simulink model "curiosity_i2c_pitch_roll"  (R2024b)
settings: Solver=FixedStepDiscrete  StartTime=0.0  StopTime=inf  FixedStep=1e-3  RelTol=1e-3  EnableMultiTasking=on
undefined symbols (not defined in the file): A0, ADC, D10, D7, D8, D9, DiscIntNeverNeededParam, Max, MaxPer, ms, NumBits1, NumBits2, P1, P58, P59, Pin, Resol, s, Timer, us
libraries: MCHP_Blockset x18, simulink x15, dspstat3 x1
(part 1 of 4)
settings Model: SimulationMode=external  ExtModeEnableFloating=off  ExtModeTrigDuration=20  Creator=I52209  LastModifiedBy=I67977
settings SolverCC: AlgebraicLoopSolver=TrustRegion
settings OptimizationCC: DefaultUnderspecifiedDataType=single  EnhancedBackFolding=on  BooleansAsBitfields=on  PassReuseOutputArgsAs=Individual arguments  ZeroExternalMemoryAtStartup=off  ZeroInternalMemoryAtStartup=off  OptimizeBlockOrder=speed  DifferentSizesBufferReuse=on  EfficientTunableParamExpr=on
settings DebuggingCC: MultiTaskDSMMsg=none  MultiTaskCondExecSysMsg=none  MultiTaskRateTransMsg=warning  ParameterTunabilityLossMsg=error  ArithmeticOperatorsInVariantConditions=warning
settings HardwareCC: ProdBitPerPointer=32  ProdBitPerSizeT=32  ProdBitPerPtrDiffT=32  ProdLargestAtomicInteger=Long  ProdWordSize=32  ProdLongLongMode=on  ProdHWDeviceType=Generic->Custom
settings ModelReferenceCC: ModelReferenceNumInstancesAllowed=Single
settings SFSimCC: MATLABDynamicMemAlloc=off  CustomCodeUndefinedFunction=UseInterfaceOnly
settings RTWCC: Description=Microchip Embedded Target dsPIC33A (real-time)  SystemTargetFile=MCHP_dsPIC33A_stf.tlc  TLCOptions="-aExtModeXCPClassicInterface=0  -aCreateExtModeTypes=1 -aExtModeXCPSimulationTimeInTicks=1"  TemplateMakefile=MCHP_dsPIC33A.tmf  GPUComputeCapability=3.5
settings CodeAppCC: ForceParamTrailComments=on  IgnoreCustomStorageClasses=off  MaxIdLength=255  OperatorAnnotations=on  SimulinkDataObjDesc=on  SFDataObjDesc=on  InsertBlockDesc=on
settings STFCustomTargetCC: TargetLibSuffix=_lib.a  TargetLangStandard=C99 (ISO)  MultiwordLength=256  CombineOutputUpdateFcns=on  CombineSignalStateStructs=on  ERTCustomFileBanners=on  SupportContinuousTime=off  RemoveResetFunc=on  MATLABClassNameForMDSCustomization=Simulink.SoftwareTarget.ERTCustomization  SystemTargetFile=MCHP_dsPIC33A_stf.tlc
settings ERTTargetCC: TargetLibSuffix=_lib.a  TargetLangStandard=C99 (ISO)  ParMdlRefBuildCompliant=off  CompOptLevelCompliant=off  ConcurrentExecutionCompliant=off  CombineSignalStateStructs=on  SupportNonInlinedSFcns=on  ModelStepFunctionPrototypeControlCompliant=off  CPPClassGenCompliant=off  UseToolchainInfoCompliant=off  ExtMode=on  ExtModeTransport=1  ExtModeStaticAlloc=on  ExtModeStaticAllocSize=2048  ExtModeMexFile=ext_xcp  ExtModeMexArgs=1 52 460800 './curiosity_i2c.X/curiosity_i2c.elf'  ExtModeIntrfLevel=Level2 - Open  InlinedParameterPlacement=Hierarchical  ERTSrcFileBannerTemplate=MCHP_dsPIC_code_template.cgt  ERTHdrFileBannerTemplate=MCHP_dsPIC_code_template.cgt  ERTDataSrcFileTemplate=MCHP_dsPIC_code_template.cgt  ERTDataHdrFileTemplate=MCHP_dsPIC_code_template.cgt  ERTCustomFileTemplate=MCHP_main.tlc  MaxLineWidth=110  DynamicArrayContainerType=coder::array

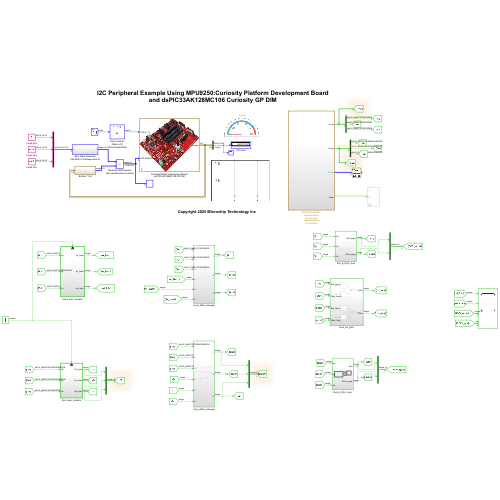
[thumbnail: Simulink's stored preview of the top-level diagram]
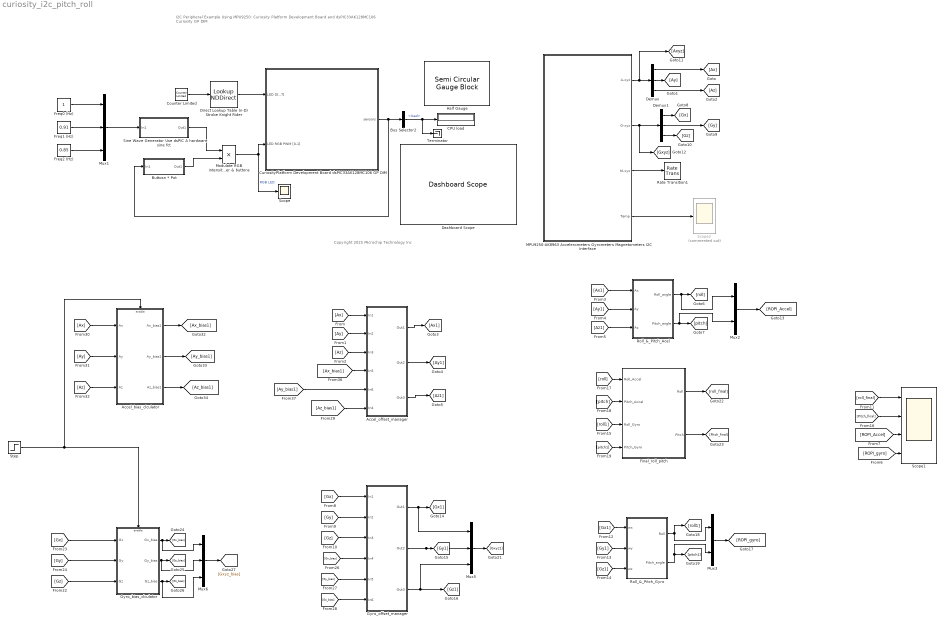
== system curiosity_i2c_pitch_roll ==
  note: I2C Peripheral Example Using MPU9250: Curiosity Platform Development Board and dsPIC33AK128MC106 Curiosity GP DIM
  note: Copyright 2025 Microchip Technology Inc
  Accel_bias_clculator : Subsystem  TreatAsAtomicUnit=on
  Accel_offset_manager : Subsystem
  Bus Selector2 : BusSelector  OutputSignals=MCU.load
  Buttosn * Pot : Subsystem
  CPU load : Display
  Counter Limited : simulink/Sources/Counter Limited  uplimit=13  tsamp=0.05
  CuriosityPlatform Development Board dsPIC33AK128MC106 GP DIM : Subsystem
      mask Display: image('MCHP_i_Board_Curiosity_dsPICA.jpg')
  Dashboard Scope : DashboardScope  TimeSpan=5  Ymin=0  Ymax=1  LegendPosition=Hide  ScaleAtStop=off  TicksPosition=Inside
  Demux : Demux  Outputs=3
  Demux1 : Demux  Outputs=3
  Direct Lookup Table (n-D) Strobe Knight Rider : LookupNDDirect  NumberOfTableDimensions=1  Table=uint16(2.^[[0:7] [6:-1:1]] )  RemoveProtectionInput=on
  Final_roll_pitch : Subsystem
  Freq0 (Hz) : Constant  OutDataTypeStr=fixdt(0,16,10)
  Freq1 (Hz) : Constant  Value=0.91  OutDataTypeStr=fixdt(0,16,10)
  Freq2 (Hz) : Constant  Value=0.85  OutDataTypeStr=fixdt(0,16,10)
  Gyro_bias_clculator : Subsystem  TreatAsAtomicUnit=on
  Gyro_offset_manager : Subsystem
  Half Gauge : SemiCircularGaugeBlock
  MPU9250-AK8963 Accelerometers Gyrometers Magnetometers I2C Interface : Subsystem
  Modulate RGB intensity with potentiometer & buttons : Product  OutDataTypeStr=single
  Mux1 : Mux  Inputs=3
  Mux2 : Mux  Inputs=2
  Mux3 : Mux  Inputs=2
  Mux5 : Mux  Inputs=3
  Mux6 : Mux  Inputs=3
  Rate Transition1 : RateTransition  Deterministic=off  OutPortSampleTimeOpt=Inherit
  Roll_&_Pitch_Acel : Subsystem
  Roll_&_Pitch_Gyro : Subsystem
  Scope : Scope
  Scope1 : Scope  NumInputPorts=4
  Scope2 : Scope  Commented=on
  Sine Wave Generator Use dsPIC A hardware sine fct : Subsystem
  Step : Step  Time=2  Before=1  After=0  SampleTime=0.005
  Terminator : Terminator
  wires:
  Buttosn * Pot/1(Out1) -> Modulate RGB intensity with potentiometer & buttons/2
  Bus Selector2/1 -> Terminator/1, CPU load/1  "<load>"
  Sine Wave Generator Use dsPIC A hardware sine fct/1(Out1) -> Modulate RGB intensity with potentiometer & buttons/1
  Mux1/1 -> Sine Wave Generator Use dsPIC A hardware sine fct/1(In1)
  Freq0 (Hz)/1 -> Mux1/1
  Freq1 (Hz)/1 -> Mux1/2
  Freq2 (Hz)/1 -> Mux1/3
  Direct Lookup Table (n-D) Strobe Knight Rider/1 -> CuriosityPlatform Development Board dsPIC33AK128MC106 GP DIM/1(LED [0...7])
  Modulate RGB intensity with potentiometer & buttons/1 -> CuriosityPlatform Development Board dsPIC33AK128MC106 GP DIM/2(LED RGB PWM [0-1]), Scope/1  "RGB LED"
  CuriosityPlatform Development Board dsPIC33AK128MC106 GP DIM/1(sensors) -> Buttosn * Pot/1(In1), Bus Selector2/1
  Counter Limited/1 -> Direct Lookup Table (n-D) Strobe Knight Rider/1
  MPU9250-AK8963 Accelerometers Gyrometers Magnetometers I2C Interface/1(A-xyz) -> Demux/1, [Axyz]
  Demux1/2 -> [Gy]
  MPU9250-AK8963 Accelerometers Gyrometers Magnetometers I2C Interface/2(G-xyz) -> [Gxyz], Demux1/1
  MPU9250-AK8963 Accelerometers Gyrometers Magnetometers I2C Interface/3(M-xyz) -> Rate Transition1/1
  MPU9250-AK8963 Accelerometers Gyrometers Magnetometers I2C Interface/4(Temp) -> Scope2/1
  Demux/1 -> [Ax]
  Demux/2 -> [Ay]
  Demux/3 -> [Az]
  Demux1/1 -> [Gx]
  Demux1/3 -> [Gz]
  [Gy] -> Gyro_offset_manager/2(In2)
  [Gy] -> Gyro_bias_clculator/2(Gy)
  Accel_offset_manager/2(Out2) -> [Ay1]
  [Ax] -> Accel_bias_clculator/1(Ax)
  Roll_&_Pitch_Acel/1(Roll_angle) -> Mux2/1, [roll]
  [Gx] -> Gyro_bias_clculator/1(Gx)
  [Ay] -> Accel_offset_manager/2(In2)
  [Az_bias1] -> Accel_offset_manager/6(In4)
  [ROPI_Accel] -> Scope1/3
  Final_roll_pitch/2(Pitch) -> [Pitch_final]
  [Ax1] -> Roll_&_Pitch_Acel/1(Ax)
  Gyro_offset_manager/2(Out2) -> Mux5/2, [Gy1]
  Mux6/1 -> [Gxyz_bias]
  [Az1] -> Roll_&_Pitch_Acel/3(Az)
  Gyro_bias_clculator/2(Gy_bias) -> Mux6/2, [Gy_bias]
  [Gx] -> Gyro_offset_manager/1(In1)
  [roll] -> Final_roll_pitch/1(Roll_Accel)
  [Az] -> Accel_offset_manager/3(In3)
  [Gz] -> Gyro_bias_clculator/3(Gz)
  [Gx1] -> Roll_&_Pitch_Gyro/1(wx)
  [roll1] -> Final_roll_pitch/3(Roll_Gyro)
  Roll_&_Pitch_Gyro/2(Pitch_angle) -> Mux3/2, [pitch1]
  Gyro_offset_manager/1(Out1) -> [Gx1], Mux5/1
  [Ay_bias1] -> Accel_offset_manager/5(In6)
  Mux2/1 -> [ROPI_Accel]
  [Gx_bias] -> Gyro_offset_manager/4(In4)
  [Ay1] -> Roll_&_Pitch_Acel/2(Ay)
  Final_roll_pitch/1(Roll) -> [roll_final]
  Step/1 -> Accel_bias_clculator/Enable, Gyro_bias_clculator/Enable
  Mux3/1 -> [ROPI_gyro]
  [pitch] -> Final_roll_pitch/2(Pitch_Accel)
  Accel_bias_clculator/2(Ay_bias1) -> [Ay_bias1]
  [Gz] -> Gyro_offset_manager/3(In3)
  Accel_bias_clculator/3(Az_bias1) -> [Az_bias1]
  Accel_offset_manager/1(Out1) -> [Ax1]
  Gyro_offset_manager/3(Out3) -> Mux5/3, [Gz1]
  Gyro_bias_clculator/1(Gx_bias) -> Mux6/1, [Gx_bias]
  [Gz_bias] -> Gyro_offset_manager/6(In6)
  [Gy1] -> Roll_&_Pitch_Gyro/2(wy)
  [Pitch_final] -> Scope1/2
  [ROPI_gyro] -> Scope1/4
  [pitch1] -> Final_roll_pitch/4(Pitch_Gyro)
  [Ay] -> Accel_bias_clculator/2(Ay)
  [Ax] -> Accel_offset_manager/1(In1)
  [roll_final] -> Scope1/1
  Mux5/1 -> [Gxyz1]
  Gyro_bias_clculator/3(Gz_bias) -> Mux6/3, [Gz_bias]
  Roll_&_Pitch_Acel/2(Pitch_angle) -> Mux2/2, [pitch]
  Accel_bias_clculator/1(Ax_bias1) -> [Ax_bias1]
  [Ax_bias1] -> Accel_offset_manager/4(In5)
  [Gy_bias] -> Gyro_offset_manager/5(In5)
  [Az] -> Accel_bias_clculator/3(Az)
  Accel_offset_manager/3(Out3) -> [Az1]
  Roll_&_Pitch_Gyro/1(Roll) -> [roll1], Mux3/1
  [Gz1] -> Roll_&_Pitch_Gyro/3(wz)

== system curiosity_i2c_pitch_roll/Accel_bias_clculator ==
  Ax : Inport
  Ay : Inport  Port=2
  Az : Inport  Port=3
  Enable : EnablePort
  manu_mean : Subsystem
  manu_mean3 : Subsystem
  manu_mean4 : Subsystem
  Ax_bias1 : Outport
  Ay_bias1 : Outport  Port=2
  Az_bias1 : Outport  Port=3
  wires:
  Ay/1 -> manu_mean3/1(Ay)
  Ax/1 -> manu_mean/1(Ax)
  Az/1 -> manu_mean4/1(Az)
  manu_mean/1(Ax_bias1) -> Ax_bias1/1
  manu_mean3/1(Ay_bias1) -> Ay_bias1/1
  manu_mean4/1(Ax_bias1) -> Az_bias1/1

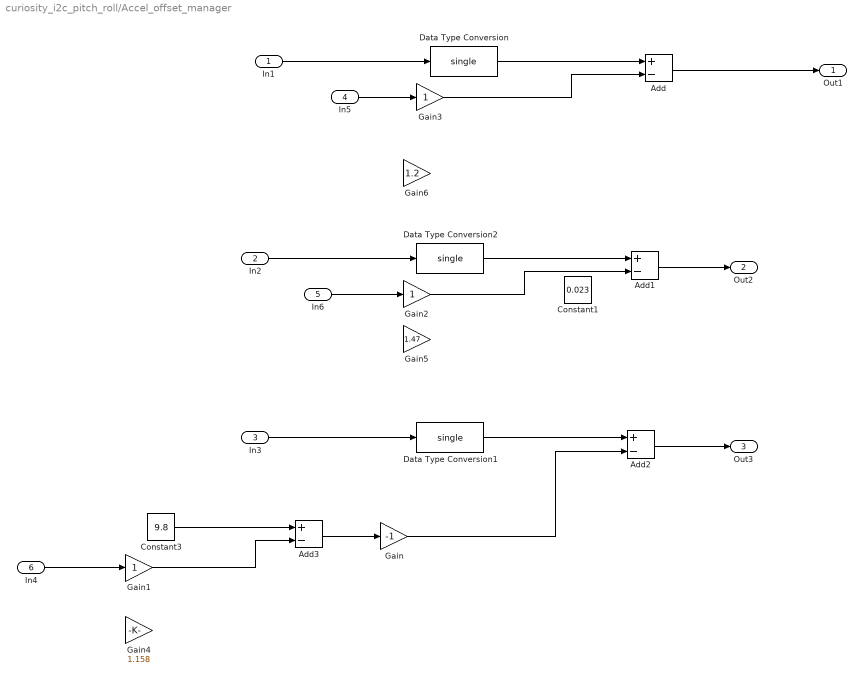
== system curiosity_i2c_pitch_roll/Accel_offset_manager ==
  In1 : Inport
  In2 : Inport  Port=2
  In3 : Inport  Port=3
  In5 : Inport  Port=4
  In6 : Inport  Port=5
  In4 : Inport  Port=6
  Add : Sum  Inputs=+-  OutDataTypeStr=Inherit: Same as first input
  Add1 : Sum  Inputs=+-  OutDataTypeStr=Inherit: Same as first input
  Add2 : Sum  Inputs=+-  OutDataTypeStr=Inherit: Same as first input
  Add3 : Sum  Inputs=+-
  Constant1 : Constant  Value=0.023  SampleTime=0.005
  Constant3 : Constant  Value=9.8  OutDataTypeStr=single  SampleTime=0.005
  Data Type Conversion : DataTypeConversion  OutDataTypeStr=single  SaturateOnIntegerOverflow=off  RndMeth=Floor
  Data Type Conversion1 : DataTypeConversion  OutDataTypeStr=single  SaturateOnIntegerOverflow=off  RndMeth=Floor
  Data Type Conversion2 : DataTypeConversion  OutDataTypeStr=single  SaturateOnIntegerOverflow=off  RndMeth=Floor
  Gain : Gain  Gain=-1
  Gain1 : Gain
  Gain2 : Gain
  Gain3 : Gain
  Gain4 : Gain  Gain=1.158
  Gain5 : Gain  Gain=1.47
  Gain6 : Gain  Gain=1.2
  Out1 : Outport
  Out2 : Outport  Port=2
  Out3 : Outport  Port=3
  wires:
  In6/1 -> Gain2/1
  Gain2/1 -> Add1/2
  Data Type Conversion2/1 -> Add1/1
  In2/1 -> Data Type Conversion2/1
  Data Type Conversion1/1 -> Add2/1
  In3/1 -> Data Type Conversion1/1
  In1/1 -> Data Type Conversion/1
  Add2/1 -> Out3/1
  Add1/1 -> Out2/1
  Data Type Conversion/1 -> Add/1
  Add/1 -> Out1/1
  Add3/1 -> Gain/1
  Constant3/1 -> Add3/1
  In4/1 -> Gain1/1
  In5/1 -> Gain3/1
  Gain3/1 -> Add/2
  Gain/1 -> Add2/2
  Gain1/1 -> Add3/2

== system curiosity_i2c_pitch_roll/Buttosn * Pot ==
  In1 : Inport
  Bus Selector : BusSelector  OutputSignals=ADC.pot
  Bus Selector1 : BusSelector  OutputSignals=BTN.S1,BTN.S2,BTN.S3
  Cast1 : DataTypeConversion  OutDataTypeStr=single  SaturateOnIntegerOverflow=off  RndMeth=Floor
  Desactivate R,G or B with buttons 1,2 or 3 multiplied by pot : Product  OutDataTypeStr=single
  Downsample x10 : Subsystem  mask{DownSample=10}
      mask prompts: DownSample "DownSample Factor"
  Mux : Mux  Inputs=3
  Rate Transition : RateTransition
  Out1 : Outport
  wires:
  Mux/1 -> Cast1/1
  Rate Transition/1 -> Desactivate R,G or B with buttons 1,2 or 3 multiplied by pot/2  "U1 CH1"
  In1/1 -> Bus Selector1/1, Bus Selector/1
  Bus Selector1/3 -> Mux/3  "<S3>"
  Downsample x10/1(Out1) -> Rate Transition/1
  Bus Selector/1 -> Downsample x10/1(In1)  "<pot>"
  Desactivate R,G or B with buttons 1,2 or 3 multiplied by pot/1 -> Out1/1
  Bus Selector1/1 -> Mux/1  "<S1>"
  Bus Selector1/2 -> Mux/2  "<S2>"
  Cast1/1 -> Desactivate R,G or B with buttons 1,2 or 3 multiplied by pot/1
